simulink model "identificacionparametrica"  (R2023b)
settings: Solver=VariableStepAuto  StartTime=0.0  StopTime=10.0  RelTol=1e-3
settings Model: Creator=lombo  LastModifiedBy=lombo

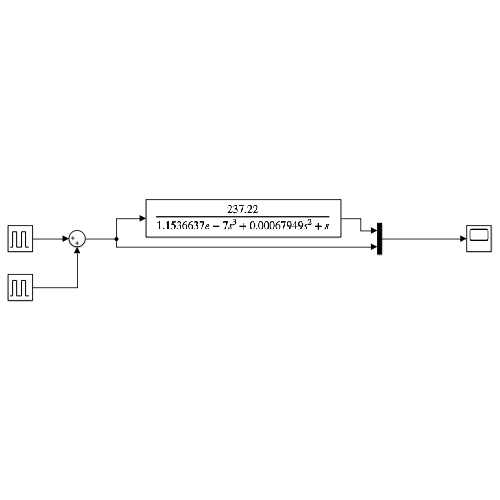
[thumbnail: Simulink's stored preview of the top-level diagram]
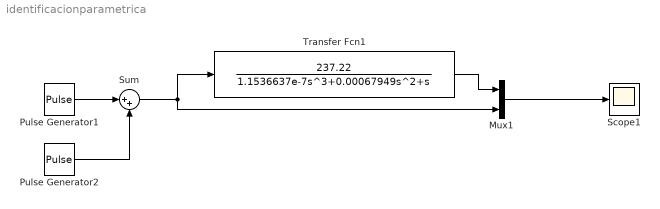
== system identificacionparametrica ==
  Mux1 : Mux  Inputs=2
  Pulse Generator1 : DiscretePulseGenerator  PulseType=Time based  Amplitude=7.04  Period=4  PulseWidth=25
  Pulse Generator2 : DiscretePulseGenerator  PulseType=Time based  Amplitude=-7.04  Period=4  PulseWidth=25  PhaseDelay=2
  Scope1 : Scope
  Sum : Sum  Inputs=|++
  Transfer Fcn1 : TransferFcn  Numerator=[237.22]  Denominator=[1.1536637e-7 0.00067949 1 0]
  wires:
  Sum/1 -> Mux1/2, Transfer Fcn1/1
  Pulse Generator1/1 -> Sum/1
  Transfer Fcn1/1 -> Mux1/1
  Pulse Generator2/1 -> Sum/2
  Mux1/1 -> Scope1/1
